simulink library "updateResponseSurface_ul"  (R2018a)
settings: Solver=VariableStepAuto  StartTime=0.0  StopTime=10.0  RelTol=1e-3
undefined symbols (not defined in the file): ctrl
libraries: createQuatraticRegressorVector x1
settings Model: Creator=mitch  LastModifiedBy=mitch

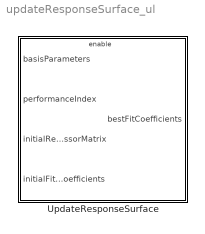
== system updateResponseSurface_ul ==
  UpdateResponseSurface : Subsystem

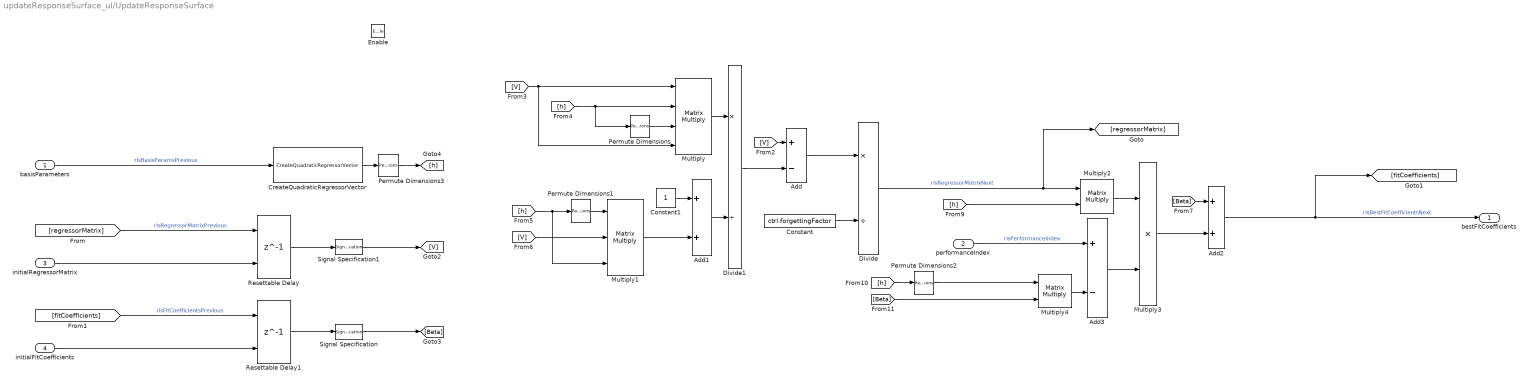
== system updateResponseSurface_ul/UpdateResponseSurface ==
  basisParameters : Inport  PortDimensions=[1 2]
  performanceIndex : Inport  Port=2
  initialRegressorMatrix : Inport  Port=3
  initialFitCoefficients : Inport  Port=4
  Enable : EnablePort
  Add : Sum  Inputs=+-
  Add1 : Sum
  Add2 : Sum
  Add3 : Sum  Inputs=+-
  Constant : Constant  Value=ctrl.forgettingFactor
  Constant1 : Constant
  CreateQuadraticRegressorVector : createQuatraticRegressorVector/CreateQuadraticRegressorVector
  Divide : Product  Inputs=*/
  Divide1 : Product  Inputs=*/
  Multiply : Product  Inputs=4  Multiplication=Matrix(*)
  Multiply1 : Product  Inputs=3  Multiplication=Matrix(*)
  Multiply2 : Product  Multiplication=Matrix(*)
  Multiply3 : Product
  Multiply4 : Product  Multiplication=Matrix(*)
  Permute Dimensions{,1..3} (4 alike) : PermuteDimensions
  Resettable Delay : Delay  DelayLength=1  InitialConditionSource=Input port
      settings: InputPortMap=u0,p4
  Resettable Delay1 : Delay  DelayLength=1  InitialConditionSource=Input port
      settings: InputPortMap=u0,p4
  Signal Specification : SignalSpecification  Dimensions=[5,1]
  Signal Specification1 : SignalSpecification  Dimensions=[5,5]
  bestFitCoefficients : Outport
  wires:
  Add2/1 -> [fitCoefficients], bestFitCoefficients/1  "rlsBestFitCoefficientsNext"
  performanceIndex/1 -> Add3/1  "rlsPerformanceIndex"
  [V] -> Multiply/4, Multiply/1
  initialRegressorMatrix/1 -> Resettable Delay/2
  initialFitCoefficients/1 -> Resettable Delay1/2
  [regressorMatrix] -> Resettable Delay/1  "rlsRegressorMatrixPrevious"
  [fitCoefficients] -> Resettable Delay1/1  "rlsFitCoefficientsPrevious"
  Constant/1 -> Divide/2
  Resettable Delay/1 -> Signal Specification1/1
  [V] -> Add/1
  Add/1 -> Divide/1
  Divide1/1 -> Add/2
  Resettable Delay1/1 -> Signal Specification/1
  Multiply/1 -> Divide1/1
  [h] -> Permute Dimensions/1, Multiply/2
  Permute Dimensions/1 -> Multiply/3
  Signal Specification/1 -> [Beta]
  Signal Specification1/1 -> [V]
  Add1/1 -> Divide1/2
  Constant1/1 -> Add1/1
  Multiply1/1 -> Add1/2
  [h] -> Multiply1/3, Permute Dimensions1/1
  Permute Dimensions1/1 -> Multiply1/1
  [V] -> Multiply1/2
  CreateQuadraticRegressorVector/1 -> Permute Dimensions3/1
  [Beta] -> Add2/1
  Divide/1 -> [regressorMatrix], Multiply2/1  "rlsRegressorMatrixNext"
  [h] -> Multiply2/2
  Multiply2/1 -> Multiply3/1
  Add3/1 -> Multiply3/2
  Multiply4/1 -> Add3/2
  [h] -> Permute Dimensions2/1
  [Beta] -> Multiply4/2
  Multiply3/1 -> Add2/2
  Permute Dimensions2/1 -> Multiply4/1
  basisParameters/1 -> CreateQuadraticRegressorVector/1  "rlsBasisParamsPrevious"
  Permute Dimensions3/1 -> [h]
